simulink model "Genna_OTRB"  (R2014a)
settings: Solver=ode3  StartTime=0.0  StopTime=5  FixedStep=.001  RelTol=1e-3
settings Model: Creator=sarahcostrell  LastModifiedBy=kothmann
settings DebuggingCC: MergeDetectMultiDrivingBlocksExec=error

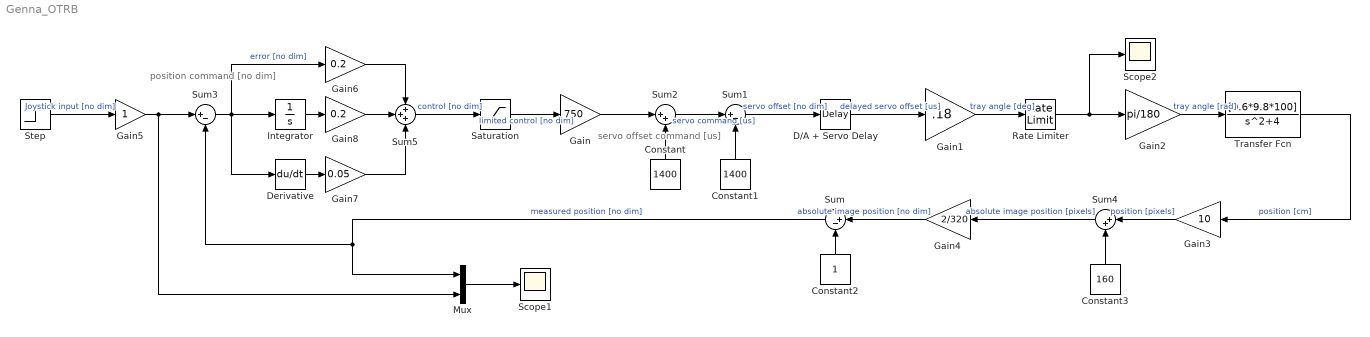
== system Genna_OTRB ==
  note: position
      | command
      | [no dim]
  note: servo
      | offset
      | command
      | [us]
  Constant : Constant  Value=1400
  Constant1 : Constant  Value=1400
  Constant2 : Constant
  Constant3 : Constant  Value=160
  D/A + Servo Delay : TransportDelay  DelayTime=.04
  Derivative : Derivative
  Gain : Gain  Gain=750
  Gain1 : Gain  Gain=.18
  Gain2 : Gain  Gain=pi/180
  Gain3 : Gain  Gain=10
  Gain4 : Gain  Gain=2/320
  Gain5 : Gain
  Gain6 : Gain  Gain=0.2
  Gain7 : Gain  Gain=0.05
  Gain8 : Gain  Gain=0.2
  Integrator : Integrator
  Mux : Mux  Inputs=2
  Rate Limiter : RateLimiter  RisingSlewLimit=1000  FallingSlewLimit=-1000  SampleTimeMode=inherited
  Saturation : Saturate
  Scope1 : Scope
      settings: TimeRange=5  YMin=0  YMax=0.7000000000000001
  Scope2 : Scope
      settings: TimeRange=5  YMin=-10  YMax=15
  Step : Step  After=.6  SampleTime=0
  Sum : Sum  Inputs=|+-
  Sum1 : Sum  Inputs=|+-
  Sum2 : Sum  Inputs=|++
  Sum3 : Sum  Inputs=|+-
  Sum4 : Sum  Inputs=|++
  Sum5 : Sum  Inputs=+++
  Transfer Fcn : TransferFcn  Numerator=[0.6*9.8*100]  Denominator=[1 0 4]
  wires:
  Sum1/1 -> D/A + Servo Delay/1  "servo offset [no dim]"
  Gain1/1 -> Rate Limiter/1  "tray angle [deg]"
  Gain2/1 -> Transfer Fcn/1  "tray angle [rad]"
  Constant1/1 -> Sum1/2
  Constant/1 -> Sum2/2
  Gain/1 -> Sum2/1
  Sum2/1 -> Sum1/1  "servo command [us]"
  Gain4/1 -> Sum/1  "absolute image position [no dim]"
  Constant2/1 -> Sum/2
  Sum5/1 -> Saturation/1  "control [no dim]"
  Sum3/1 -> Derivative/1, Integrator/1, Gain6/1  "error [no dim]"
  Gain5/1 -> Mux/2, Sum3/1
  Step/1 -> Gain5/1  "Joystick input [no dim]"
  Saturation/1 -> Gain/1  "limited control [no dim]"
  Transfer Fcn/1 -> Gain3/1  "position [cm]"
  Constant3/1 -> Sum4/2
  Gain3/1 -> Sum4/1  "position [pixels]"
  D/A + Servo Delay/1 -> Gain1/1  "delayed servo offset [us]"
  Sum4/1 -> Gain4/1  "absolute image position [pixels]"
  Sum/1 -> Sum3/2, Mux/1  "measured position [no dim]"
  Mux/1 -> Scope1/1
  Derivative/1 -> Gain7/1
  Gain6/1 -> Sum5/1
  Integrator/1 -> Gain8/1
  Gain8/1 -> Sum5/2
  Gain7/1 -> Sum5/3
  Rate Limiter/1 -> Scope2/1, Gain2/1
